simulink model "Ej1"  (R2023a)
settings: Solver=VariableStepAuto  StartTime=0.0  StopTime=20  RelTol=1e-3
settings Model: Creator=santi  LastModifiedBy=santi

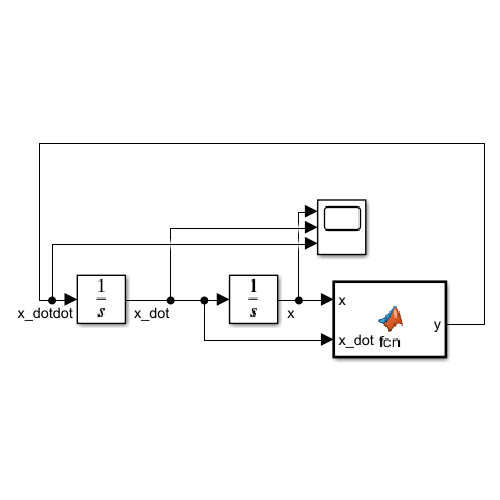
[thumbnail: Simulink's stored preview of the top-level diagram]
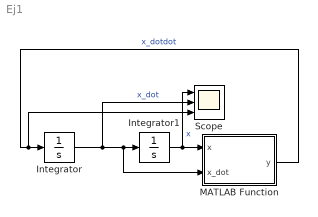
== system Ej1 ==
  Integrator : Integrator  InitialCondition=0.25
  Integrator1 : Integrator  InitialCondition=1
  MATLAB Function : MATLAB Function  TreatAsAtomicUnit=on
  Scope : Scope  NumInputPorts=3
  wires:
  Integrator/1 -> Scope/2, MATLAB Function/2(x_dot), Integrator1/1  "x_dot"
  MATLAB Function/1(y) -> Scope/3, Integrator/1  "x_dotdot"
  Integrator1/1 -> Scope/1, MATLAB Function/1(x)  "x"

== matlab function Ej1/MATLAB Function ==
  data: x input; y output; x_dot input
function y = fcn(x, x_dot)

y = -1*((x^2-1)*x_dot+x);
